simulink model "inner_chamber"  (R2025b)
settings: Solver=FixedStepAuto  StartTime=0.0  StopTime=10.0  FixedStep=0.001  RelTol=1e-3
settings Model: Creator=vasilisgkionis  LastModifiedBy=vasilisgkionis

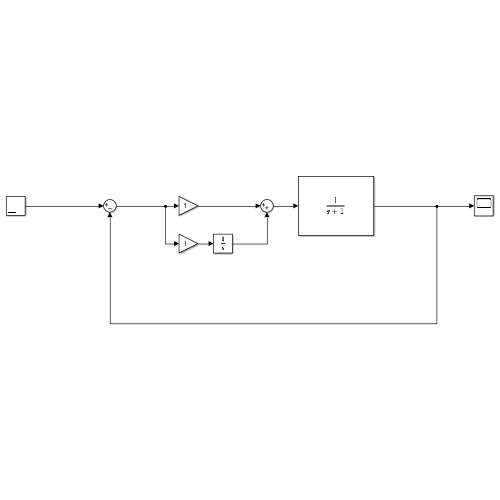
[thumbnail: Simulink's stored preview of the top-level diagram]
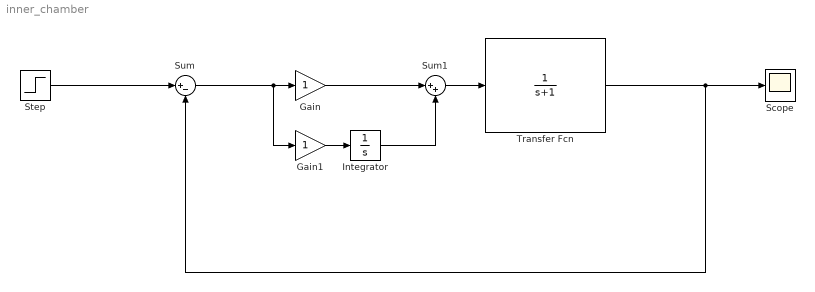
== system inner_chamber ==
  Gain : Gain
  Gain1 : Gain
  Integrator : Integrator
  Scope : Scope
  Step : Step  SampleTime=0
  Sum : Sum  Inputs=|+-
  Sum1 : Sum  Inputs=|++
  Transfer Fcn : TransferFcn  Denominator=[1 1]
  wires:
  Transfer Fcn/1 -> Sum/2, Scope/1
  Step/1 -> Sum/1
  Sum/1 -> Gain/1, Gain1/1
  Integrator/1 -> Sum1/2
  Gain1/1 -> Integrator/1
  Gain/1 -> Sum1/1
  Sum1/1 -> Transfer Fcn/1
